simulink model "untitled"  (R2017a)
settings: Solver=VariableStepAuto  StartTime=0.0  StopTime=10.0  RelTol=1e-3
settings Model: Creator=DoktorHax  LastModifiedBy=DoktorHax

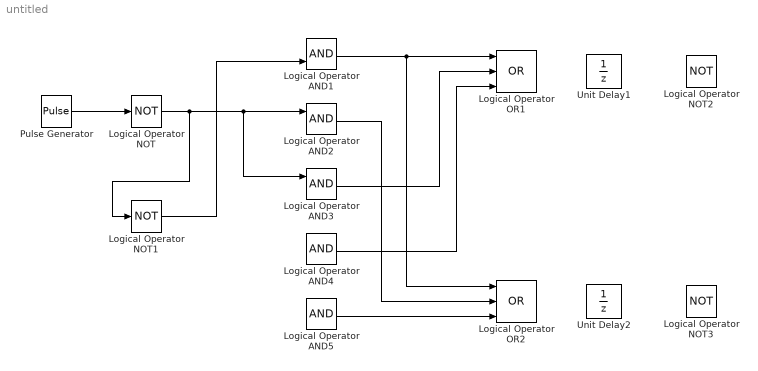
== system untitled ==
  Logical Operator AND{1..5} (5 alike) : Logic  AllPortsSameDT=off  OutDataTypeStr=boolean
  Logical Operator NOT{,1..3} (4 alike) : Logic  Operator=NOT  AllPortsSameDT=off  OutDataTypeStr=boolean
  Logical Operator OR1 : Logic  Operator=OR  Inputs=3  AllPortsSameDT=off  OutDataTypeStr=boolean
  Logical Operator OR2 : Logic  Operator=OR  Inputs=3  AllPortsSameDT=off  OutDataTypeStr=boolean
  Pulse Generator : DiscretePulseGenerator  PulseType=Time based  Period=10  PulseWidth=5
  Unit Delay1 : UnitDelay  SampleTime=-1
  Unit Delay2 : UnitDelay  SampleTime=-1
  wires:
  Pulse Generator/1 -> Logical Operator NOT/1
  Logical Operator NOT/1 -> Logical Operator NOT1/1, Logical Operator AND2/1, Logical Operator AND3/1
  Logical Operator NOT1/1 -> Logical Operator AND1/2
  Logical Operator AND1/1 -> Logical Operator OR1/1, Logical Operator OR2/1
  Logical Operator AND3/1 -> Logical Operator OR1/2
  Logical Operator AND4/1 -> Logical Operator OR1/3
  Logical Operator AND2/1 -> Logical Operator OR2/2
  Logical Operator AND5/1 -> Logical Operator OR2/3
